simulink model "L1_C"  (R2020a)
settings: Solver=VariableStepAuto  StartTime=0.0  StopTime=10.0  RelTol=1e-3
settings Model: Creator=fbi  LastModifiedBy=fbi

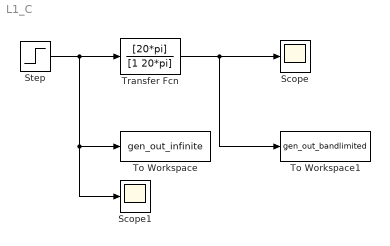
== system L1_C ==
  Scope : Scope
  Scope1 : Scope
  Step : Step  Time=0  SampleTime=0
  To Workspace : ToWorkspace  VariableName=gen_out_infinite  SampleTime=-1
  To Workspace1 : ToWorkspace  VariableName=gen_out_bandlimited  SampleTime=-1
  Transfer Fcn : TransferFcn  Numerator=[20*pi]  Denominator=[1 20*pi]
  wires:
  Step/1 -> Scope1/1, To Workspace/1, Transfer Fcn/1
  Transfer Fcn/1 -> To Workspace1/1, Scope/1
